simulink model "DiscretizedModel"  (R2023b)
settings: Solver=VariableStepAuto  StartTime=0.0  StopTime=0.5  MaxStep=inverter.param.timeSwitching*0.1  RelTol=1e-3
undefined symbols (not defined in the file or in its folder): contr_D, contr_Q, contr_W, inverter, mot
libraries: eeGeneralControl x1
settings Model: Creator=zambo  LastModifiedBy=zambo

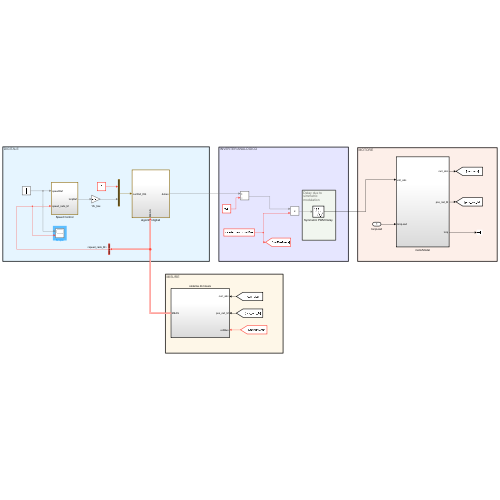
[thumbnail: Simulink's stored preview of the top-level diagram]
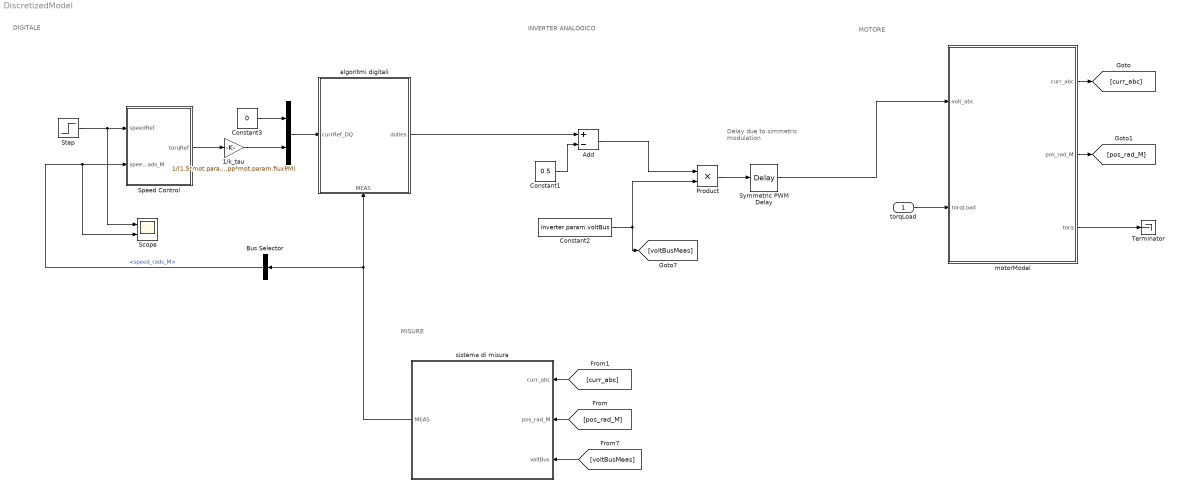
== system DiscretizedModel ==
  note: MISURE
  note: MOTORE
  note: DIGITALE
  note: INVERTER ANALOGICO
  note: Delay due to
      | simmetric
      | modulation
  torqLoad : Inport
  1/k_tau : Gain  Gain=1/(1.5*mot.param.pp*mot.param.fluxPM)
  Add : Sum  Inputs=+-
  Bus Selector : BusSelector  OutputSignals=speed.speed_rads_M
  Constant1 : Constant  Value=0.5  SampleTime=inverter.param.timeSampling
  Constant2 : Constant  Value=inverter.param.voltBus  SampleTime=inverter.param.timeSampling
  Constant3 : Constant  Value=0  SampleTime=inverter.param.timeSampling
  Mux : Mux  Inputs=2
  Product : Product
  Scope : Scope  NumInputPorts=2
  Speed Control : Subsystem
  Step : Step  Time=0.2  After=280  SampleTime=0
  Symmetric PWM Delay : TransportDelay  DelayTime=inverter.param.timeSwitching*0.5
  Terminator : Terminator
  algoritmi digitali : Subsystem
      settings: PortSchema="{\"entries\":[{\"content\":{\"sides\":[{\"content\":{\"connectorIds\":[\"In1\"]},\"type\":\"ConnectorPlacement.EquallySpacedRectSide\",\"uuid\":\"be98b178-87c5-4194-8b79-c3f3cfcc0fc0\"},{\"content\":{\"connectorIds\":[\"Out1\"],\"side\":\"RIGHT\"},\"type\":\"ConnectorPlacement.EquallySpacedRectSide\",\"uuid\":\"8217c3eb-ba2e-412f-a9c4-f2e3b7cd9b00\"},{\"content\":{\"side\":\"TOP\"},\"type\":\"ConnectorPlacement.EquallySpacedRectSide\",\"uuid\":\"9b7fad55-3d61-41f3-9dee-47d3dc8a32f9\"},{\"content\":{\"connectorIds\":[\"In2\"],\"side\":\"BOTTOM\"},\"type\":\"ConnectorPlacement.EquallySpacedRectSide\",\"uuid\":\"8ebbf679-530e-4b8b-8dca-2f31264a1f1b\"}]},\"type\":\"ConnectorPlacement.EquallySpacedConnector\",\"uuid\":\"25d4c349-4b88-4de2-b9c1-687bdffd88d1\"}],\"packageUris\":[\"http://schema.mathworks.com/mf0/Connector/R2020b\"],\"version\":\"1.0\"}"
  motorModel : Subsystem
  sistema di misura : Subsystem
  wires:
  Bus Selector/1 -> Scope/2, Speed Control/2(speed_rads_M)  "<speed_rads_M>"
  Mux/1 -> algoritmi digitali/1(currRef_DQ)
  [pos_rad_M] -> sistema di misura/2(pos_rad_M)
  motorModel/3(torq) -> Terminator/1
  sistema di misura/1(MEAS) -> Bus Selector/1, algoritmi digitali/2(MEAS)
  Step/1 -> Scope/1, Speed Control/1(speedRef)
  [curr_abc] -> sistema di misura/1(curr_abc)
  motorModel/2(pos_rad_M) -> [pos_rad_M]
  Constant1/1 -> Add/2
  Symmetric PWM Delay/1 -> motorModel/1(volt_abc)
  Speed Control/1(torqRef) -> 1/k_tau/1
  Add/1 -> Product/1
  Product/1 -> Symmetric PWM Delay/1
  motorModel/1(curr_abc) -> [curr_abc]
  Constant3/1 -> Mux/1
  algoritmi digitali/1(duties) -> Add/1
  Constant2/1 -> Product/2, [voltBusMeas]
  1/k_tau/1 -> Mux/2
  [voltBusMeas] -> sistema di misura/3(voltBus)
  torqLoad/1 -> motorModel/2(torqLoad)

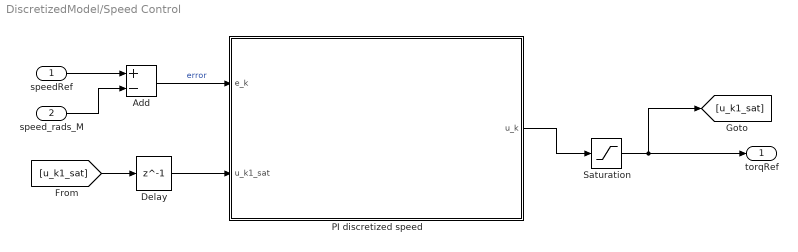
== system DiscretizedModel/Speed Control ==
  speedRef : Inport
  speed_rads_M : Inport  Port=2
  Add : Sum  Inputs=+-
  Delay : Delay  DelayLength=1
  PI discretized speed : MATLAB Function  TreatAsAtomicUnit=on
  Saturation : Saturate  UpperLimit=0.22  LowerLimit=-0.22
  torqRef : Outport
  wires:
  speedRef/1 -> Add/1
  speed_rads_M/1 -> Add/2
  Saturation/1 -> [u_k1_sat], torqRef/1
  Add/1 -> PI discretized speed/1(e_k)  "error"
  PI discretized speed/1(u_k) -> Saturation/1
  [u_k1_sat] -> Delay/1
  Delay/1 -> PI discretized speed/2(u_k1_sat)

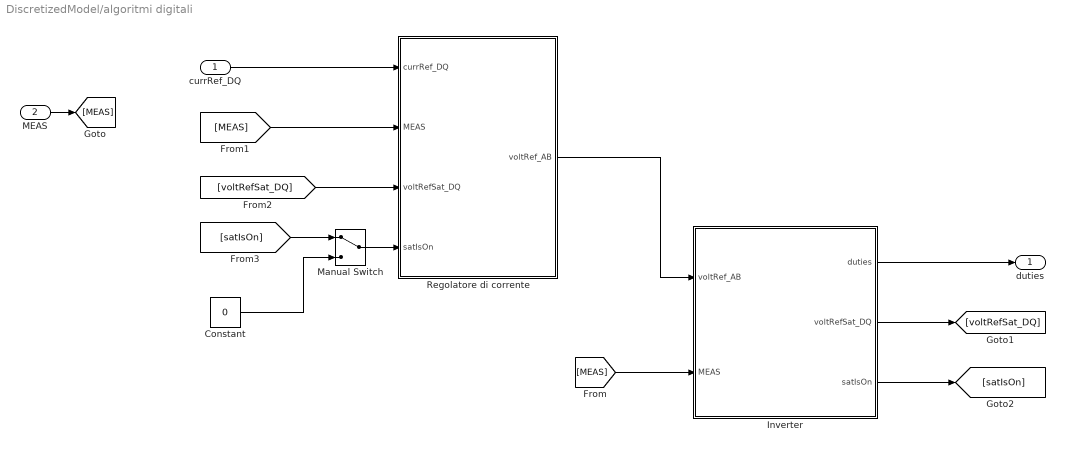
== system DiscretizedModel/algoritmi digitali ==
  currRef_DQ : Inport
  MEAS : Inport  Port=2
  Constant : Constant  Value=0  SampleTime=inverter.param.timeSampling
  Inverter : Subsystem
  Manual Switch : ManualSwitch
  Regolatore di corrente : Subsystem
  duties : Outport
  wires:
  Inverter/1(duties) -> duties/1
  MEAS/1 -> [MEAS]
  [MEAS] -> Inverter/2(MEAS)
  currRef_DQ/1 -> Regolatore di corrente/1(currRef_DQ)
  Regolatore di corrente/1(voltRef_AB) -> Inverter/1(voltRef_AB)
  Inverter/3(satIsOn) -> [satIsOn]
  [MEAS] -> Regolatore di corrente/2(MEAS)
  Inverter/2(voltRefSat_DQ) -> [voltRefSat_DQ]
  [voltRefSat_DQ] -> Regolatore di corrente/3(voltRefSat_DQ)
  Manual Switch/1 -> Regolatore di corrente/4(satIsOn)
  Constant/1 -> Manual Switch/2
  [satIsOn] -> Manual Switch/1

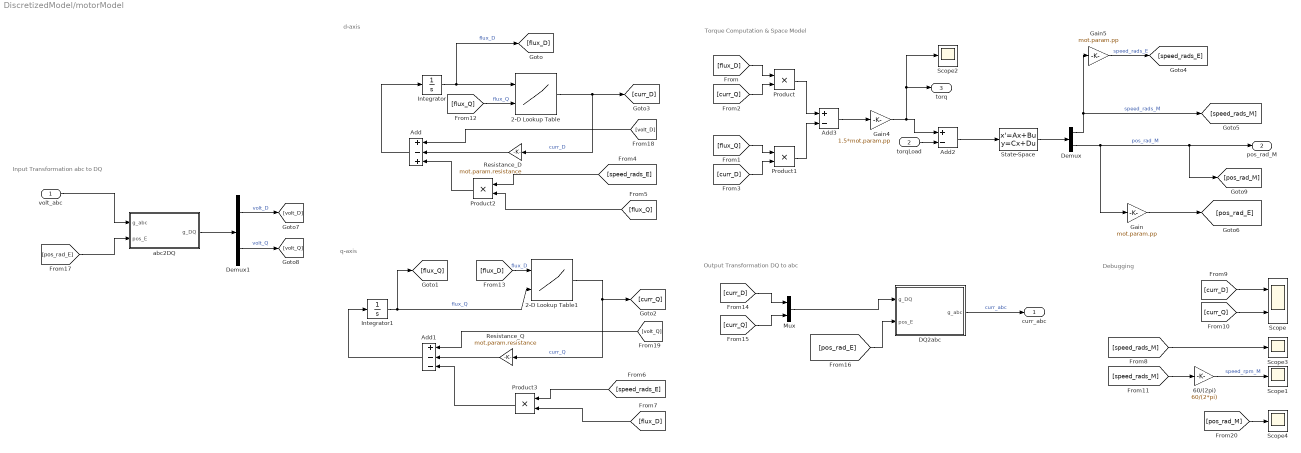
== system DiscretizedModel/motorModel ==
  note: q-axis
  note: d-axis
  note: Debugging
  note: Torque Computation & Space Model
  note: Output Transformation DQ to abc
  note: Input Transformation abc to DQ
  volt_abc : Inport
  torqLoad : Inport  Port=2
  2-D Lookup Table : Lookup_n-D  BreakpointsForDimension1=mot.maps.fluxVec_D  BreakpointsForDimension2=mot.maps.fluxVec_Q  Table=mot.maps.currMap_D'  InternalRulePriority=Speed  RndMeth=Simplest
      settings: InputPortMap=u0,u1
  2-D Lookup Table1 : Lookup_n-D  BreakpointsForDimension1=mot.maps.fluxVec_D  BreakpointsForDimension2=mot.maps.fluxVec_Q  Table=mot.maps.currMap_Q'  InternalRulePriority=Speed  RndMeth=Simplest
      settings: InputPortMap=u0,u1
  60/(2pi) : Gain  Gain=60/(2*pi)
  Add : Sum  Inputs=+-+
  Add1 : Sum  Inputs=+--
  Add2 : Sum  Inputs=+-
  Add3 : Sum  Inputs=+-
  DQ2abc : MATLAB Function  TreatAsAtomicUnit=on
  Demux : Demux  Outputs=2
  Demux1 : Demux  Outputs=2
  Gain : Gain  Gain=mot.param.pp
  Gain4 : Gain  Gain=1.5*mot.param.pp
  Gain5 : Gain  Gain=mot.param.pp
  Integrator : Integrator  InitialCondition=mot.param.fluxPM
  Integrator1 : Integrator
  Mux : Mux  Inputs=2
  Product{,1..3} (4 alike) : Product
  Resistance_D : Gain  Gain=mot.param.resistance
  Resistance_Q : Gain  Gain=mot.param.resistance
  Scope : Scope  NumInputPorts=2
  Scope{1..4} (4 alike) : Scope
  State-Space : StateSpace  A=mot.param.Amech  B=mot.param.Bmech  C=mot.param.Cmech  D=mot.param.Dmech  InitialCondition=[0 0]
  abc2DQ : MATLAB Function  TreatAsAtomicUnit=on
  curr_abc : Outport
  pos_rad_M : Outport  Port=2
  torq : Outport  Port=3
  wires:
  [volt_Q] -> Add1/1
  [flux_Q] -> 2-D Lookup Table/2  "flux_Q"
  [speed_rads_M] -> Scope3/1
  Gain/1 -> [pos_rad_E]
  Integrator/1 -> 2-D Lookup Table/1, [flux_D]  "flux_D"
  [curr_D] -> Mux/1
  Demux1/2 -> [volt_Q]  "volt_Q"
  [pos_rad_E] -> abc2DQ/2(pos_E)
  [curr_Q] -> Product/2
  abc2DQ/1(g_DQ) -> Demux1/1
  Resistance_Q/1 -> Add1/2
  [curr_Q] -> Mux/2
  Product3/1 -> Add1/3
  [pos_rad_E] -> DQ2abc/2(pos_E)
  Demux1/1 -> [volt_D]  "volt_D"
  [flux_D] -> Product3/2
  [speed_rads_E] -> Product2/1
  Demux/2 -> Gain/1, [pos_rad_M], pos_rad_M/1  "pos_rad_M"
  Product2/1 -> Add/3
  [speed_rads_E] -> Product3/1
  Product/1 -> Add3/1
  Add1/1 -> Integrator1/1
  DQ2abc/1(g_abc) -> curr_abc/1  "curr_abc"
  2-D Lookup Table/1 -> Resistance_D/1, [curr_D]  "curr_D"
  Add3/1 -> Gain4/1
  [curr_D] -> Product1/2
  [flux_D] -> Product/1
  Add/1 -> Integrator/1
  Product1/1 -> Add3/2
  volt_abc/1 -> abc2DQ/1(g_abc)
  Integrator1/1 -> 2-D Lookup Table1/2, [flux_Q]  "flux_Q"
  Demux/1 -> [speed_rads_M], Gain5/1  "speed_rads_M"
  [pos_rad_M] -> Scope4/1
  Gain4/1 -> torq/1, Scope2/1, Add2/1
  [speed_rads_M] -> 60/(2pi)/1
  Gain5/1 -> [speed_rads_E]  "speed_rads_E"
  Resistance_D/1 -> Add/2
  2-D Lookup Table1/1 -> Resistance_Q/1, [curr_Q]  "curr_Q"
  60/(2pi)/1 -> Scope1/1  "speed_rpm_M"
  [volt_D] -> Add/1
  [flux_Q] -> Product2/2
  Mux/1 -> DQ2abc/1(g_DQ)
  [curr_D] -> Scope/1
  [flux_Q] -> Product1/1
  State-Space/1 -> Demux/1
  [flux_D] -> 2-D Lookup Table1/1  "flux_D"
  [curr_Q] -> Scope/2
  Add2/1 -> State-Space/1
  torqLoad/1 -> Add2/2

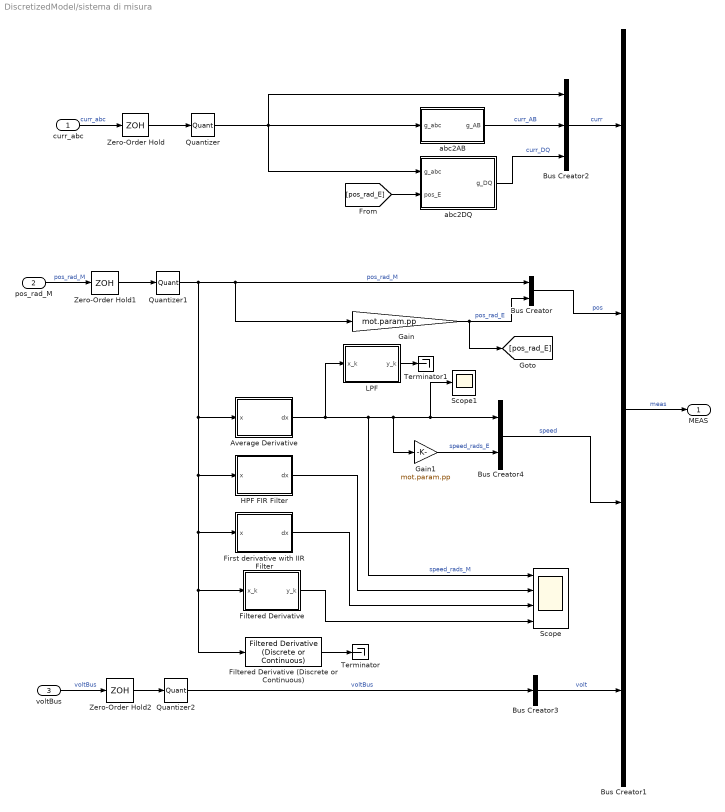
== system DiscretizedModel/sistema di misura ==
  curr_abc : Inport
  pos_rad_M : Inport  Port=2
  voltBus : Inport  Port=3
  Average Derivative : MATLAB Function  TreatAsAtomicUnit=on
  Bus Creator : BusCreator  Inputs=2
  Bus Creator1 : BusCreator  Inputs=4
  Bus Creator2 : BusCreator  Inputs=3
  Bus Creator3 : BusCreator  Inputs=1
  Bus Creator4 : BusCreator  Inputs=2
  Filtered Derivative : MATLAB Function  TreatAsAtomicUnit=on
  Filtered Derivative (Discrete or Continuous) : eeGeneralControl/Filtered Derivative (Discrete or Continuous)  K=1  T=3.9809e-04  B=inf  A=-inf  minRatio=10  init_option=Inherited from block input  x0=0  Ts=inverter.param.timeSampling
      settings: LibrarySourceBlock=|
      | ee_sl_lib/General Control/Filtered Derivative
      | (Discrete or Continuous)
  First derivative with IIR Filter : MATLAB Function  TreatAsAtomicUnit=on
  Gain : Gain  Gain=mot.param.pp
  Gain1 : Gain  Gain=mot.param.pp
  HPF FIR Filter : MATLAB Function  TreatAsAtomicUnit=on
  LPF : MATLAB Function  TreatAsAtomicUnit=on
  Quantizer : Quantizer  QuantizationInterval=meas.quant.currMeas
  Quantizer1 : Quantizer  QuantizationInterval=meas.quant.currMeas
  Quantizer2 : Quantizer  QuantizationInterval=meas.quant.currMeas
  Scope : Scope  NumInputPorts=4
  Scope1 : Scope
  Terminator : Terminator
  Terminator1 : Terminator
  Zero-Order Hold : ZeroOrderHold  SampleTime=inverter.param.timeSampling
  Zero-Order Hold1 : ZeroOrderHold  SampleTime=inverter.param.timeSampling
  Zero-Order Hold2 : ZeroOrderHold  SampleTime=inverter.param.timeSampling
  abc2AB : MATLAB Function  TreatAsAtomicUnit=on
  abc2DQ : MATLAB Function  TreatAsAtomicUnit=on
  MEAS : Outport
  wires:
  Bus Creator2/1 -> Bus Creator1/1  "curr"
  pos_rad_M/1 -> Zero-Order Hold1/1  "pos_rad_M"
  abc2DQ/1(g_DQ) -> Bus Creator2/3  "curr_DQ"
  Gain/1 -> [pos_rad_E], Bus Creator/2  "pos_rad_E"
  Quantizer1/1 -> Filtered Derivative (Discrete or Continuous)/1, Filtered Derivative/1(x_k), First derivative with IIR Filter/1(x), HPF FIR Filter/1(x), Average Derivative/1(x), Gain/1, Bus Creator/1  "pos_rad_M"
  Gain1/1 -> Bus Creator4/2  "speed_rads_E"
  Bus Creator4/1 -> Bus Creator1/3  "speed"
  Zero-Order Hold1/1 -> Quantizer1/1
  curr_abc/1 -> Zero-Order Hold/1  "curr_abc"
  [pos_rad_E] -> abc2DQ/2(pos_E)
  Zero-Order Hold/1 -> Quantizer/1
  Bus Creator1/1 -> MEAS/1  "meas"
  Bus Creator/1 -> Bus Creator1/2  "pos"
  Bus Creator3/1 -> Bus Creator1/4  "volt"
  abc2AB/1(g_AB) -> Bus Creator2/2  "curr_AB"
  Quantizer/1 -> abc2DQ/1(g_abc), Bus Creator2/1, abc2AB/1(g_abc)
  Average Derivative/1(dx) -> LPF/1(x_k), Scope1/1, Bus Creator4/1, Gain1/1, Scope/1  "speed_rads_M"
  Zero-Order Hold2/1 -> Quantizer2/1
  voltBus/1 -> Zero-Order Hold2/1  "voltBus"
  Quantizer2/1 -> Bus Creator3/1  "voltBus"
  First derivative with IIR Filter/1(dx) -> Scope/3
  HPF FIR Filter/1(dx) -> Scope/2
  Filtered Derivative/1(y_k) -> Scope/4
  Filtered Derivative (Discrete or Continuous)/1 -> Terminator/1
  LPF/1(y_k) -> Terminator1/1

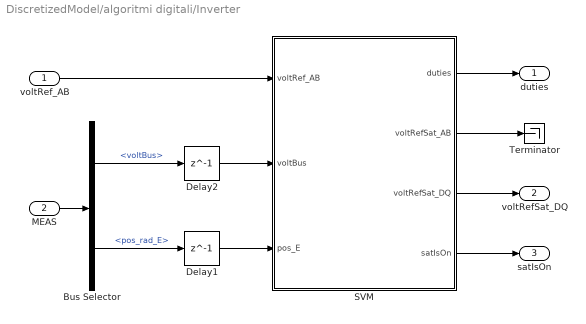
== system DiscretizedModel/algoritmi digitali/Inverter ==
  voltRef_AB : Inport
  MEAS : Inport  Port=2
  Bus Selector : BusSelector  OutputSignals=volt.voltBus,pos.pos_rad_E
  Delay1 : Delay  DelayLength=1
  Delay2 : Delay  DelayLength=1
  SVM : MATLAB Function  TreatAsAtomicUnit=on
  Terminator : Terminator
  duties : Outport
  voltRefSat_DQ : Outport  Port=2
  satIsOn : Outport  Port=3
  wires:
  Bus Selector/2 -> Delay1/1  "<pos_rad_E>"
  Delay1/1 -> SVM/3(pos_E)
  Delay2/1 -> SVM/2(voltBus)
  Bus Selector/1 -> Delay2/1  "<voltBus>"
  MEAS/1 -> Bus Selector/1
  voltRef_AB/1 -> SVM/1(voltRef_AB)
  SVM/1(duties) -> duties/1
  SVM/2(voltRefSat_AB) -> Terminator/1
  SVM/3(voltRefSat_DQ) -> voltRefSat_DQ/1
  SVM/4(satIsOn) -> satIsOn/1

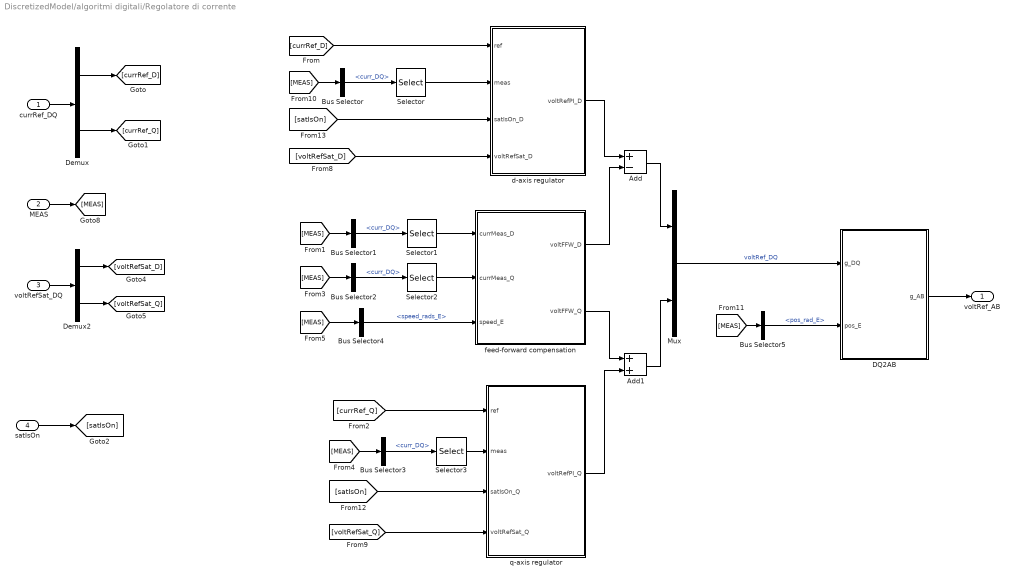
== system DiscretizedModel/algoritmi digitali/Regolatore di corrente ==
  currRef_DQ : Inport
  MEAS : Inport  Port=2
  voltRefSat_DQ : Inport  Port=3
  satIsOn : Inport  Port=4
  Add : Sum  Inputs=+-
  Add1 : Sum
  Bus Selector{,1..3} (4 alike) : BusSelector  OutputSignals=curr.curr_DQ
  Bus Selector4 : BusSelector  OutputSignals=speed.speed_rads_E
  Bus Selector5 : BusSelector  OutputSignals=pos.pos_rad_E
  DQ2AB : MATLAB Function  TreatAsAtomicUnit=on
  Demux : Demux  Outputs=2
  Demux2 : Demux  Outputs=2
  Mux : Mux  Inputs=2
  Selector : Selector  InputPortWidth=2  IndexOptions=Index vector (dialog)  Indices=[1]  OutputSizes=1
  Selector1 : Selector  InputPortWidth=2  IndexOptions=Index vector (dialog)  Indices=[1]  OutputSizes=1
  Selector2 : Selector  InputPortWidth=2  IndexOptions=Index vector (dialog)  Indices=[2]  OutputSizes=1
  Selector3 : Selector  InputPortWidth=2  IndexOptions=Index vector (dialog)  Indices=[2]  OutputSizes=1
  d-axis regulator : Subsystem
  feed-forward compensation : Subsystem
  q-axis regulator : Subsystem
  voltRef_AB : Outport
  wires:
  currRef_DQ/1 -> Demux/1
  voltRefSat_DQ/1 -> Demux2/1
  Demux/1 -> [currRef_D]
  Demux/2 -> [currRef_Q]
  [currRef_D] -> d-axis regulator/1(ref)
  [currRef_Q] -> q-axis regulator/1(ref)
  d-axis regulator/1(voltRefPI_D) -> Add/1
  feed-forward compensation/1(voltFFW_D) -> Add/2
  feed-forward compensation/2(voltFFW_Q) -> Add1/1
  q-axis regulator/1(voltRefPI_Q) -> Add1/2
  Add1/1 -> Mux/2
  Add/1 -> Mux/1
  Demux2/1 -> [voltRefSat_D]
  Demux2/2 -> [voltRefSat_Q]
  [voltRefSat_D] -> d-axis regulator/4(voltRefSat_D)
  [voltRefSat_Q] -> q-axis regulator/4(voltRefSat_Q)
  Mux/1 -> DQ2AB/1(g_DQ)  "voltRef_DQ"
  DQ2AB/1(g_AB) -> voltRef_AB/1
  MEAS/1 -> [MEAS]
  [MEAS] -> Bus Selector/1
  Bus Selector/1 -> Selector/1  "<curr_DQ>"
  Selector/1 -> d-axis regulator/2(meas)
  Bus Selector1/1 -> Selector1/1  "<curr_DQ>"
  [MEAS] -> Bus Selector1/1
  Selector1/1 -> feed-forward compensation/1(currMeas_D)
  [MEAS] -> Bus Selector2/1
  Bus Selector2/1 -> Selector2/1  "<curr_DQ>"
  Selector2/1 -> feed-forward compensation/2(currMeas_Q)
  Bus Selector3/1 -> Selector3/1  "<curr_DQ>"
  [MEAS] -> Bus Selector3/1
  Selector3/1 -> q-axis regulator/2(meas)
  [MEAS] -> Bus Selector4/1
  Bus Selector4/1 -> feed-forward compensation/3(speed_E)  "<speed_rads_E>"
  [MEAS] -> Bus Selector5/1
  Bus Selector5/1 -> DQ2AB/2(pos_E)  "<pos_rad_E>"
  satIsOn/1 -> [satIsOn]
  [satIsOn] -> q-axis regulator/3(satIsOn_Q)
  [satIsOn] -> d-axis regulator/3(satIsOn_D)

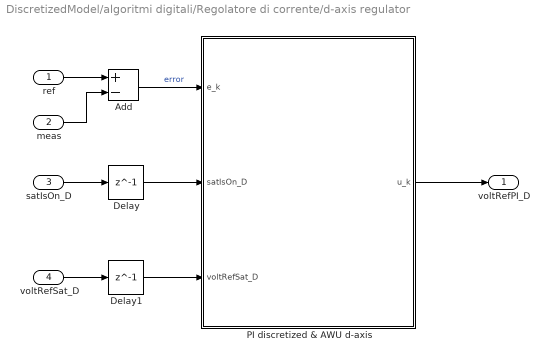
== system DiscretizedModel/algoritmi digitali/Regolatore di corrente/d-axis regulator ==
  ref : Inport
  meas : Inport  Port=2
  satIsOn_D : Inport  Port=3
  voltRefSat_D : Inport  Port=4
  Add : Sum  Inputs=+-
  Delay : Delay  DelayLength=1
  Delay1 : Delay  DelayLength=1
  PI discretized & AWU d-axis : MATLAB Function  TreatAsAtomicUnit=on
  voltRefPI_D : Outport
  wires:
  meas/1 -> Add/2
  ref/1 -> Add/1
  satIsOn_D/1 -> Delay/1
  voltRefSat_D/1 -> Delay1/1
  Add/1 -> PI discretized & AWU d-axis/1(e_k)  "error"
  Delay/1 -> PI discretized & AWU d-axis/2(satIsOn_D)
  Delay1/1 -> PI discretized & AWU d-axis/3(voltRefSat_D)
  PI discretized & AWU d-axis/1(u_k) -> voltRefPI_D/1

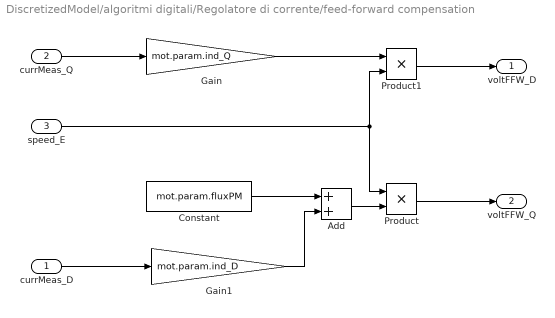
== system DiscretizedModel/algoritmi digitali/Regolatore di corrente/feed-forward compensation ==
  currMeas_D : Inport
  currMeas_Q : Inport  Port=2
  speed_E : Inport  Port=3
  Add : Sum
  Constant : Constant  Value=mot.param.fluxPM
  Gain : Gain  Gain=mot.param.ind_Q
  Gain1 : Gain  Gain=mot.param.ind_D
  Product : Product
  Product1 : Product
  voltFFW_D : Outport
  voltFFW_Q : Outport  Port=2
  wires:
  currMeas_D/1 -> Gain1/1
  currMeas_Q/1 -> Gain/1
  Constant/1 -> Add/1
  Gain1/1 -> Add/2
  Add/1 -> Product/2
  speed_E/1 -> Product/1, Product1/2
  Gain/1 -> Product1/1
  Product1/1 -> voltFFW_D/1
  Product/1 -> voltFFW_Q/1

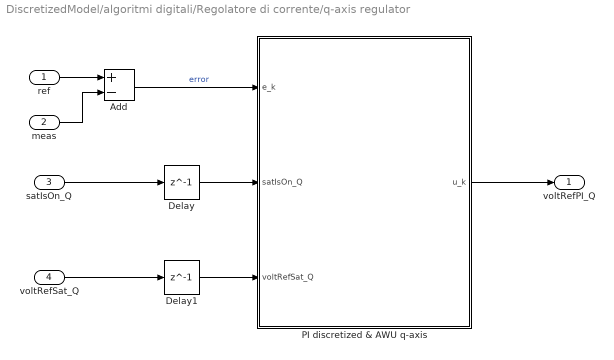
== system DiscretizedModel/algoritmi digitali/Regolatore di corrente/q-axis regulator ==
  ref : Inport
  meas : Inport  Port=2
  satIsOn_Q : Inport  Port=3
  voltRefSat_Q : Inport  Port=4
  Add : Sum  Inputs=+-
  Delay : Delay  DelayLength=1
  Delay1 : Delay  DelayLength=1
  PI discretized & AWU q-axis : MATLAB Function  TreatAsAtomicUnit=on
  voltRefPI_Q : Outport
  wires:
  ref/1 -> Add/1
  meas/1 -> Add/2
  Delay/1 -> PI discretized & AWU q-axis/2(satIsOn_Q)
  Delay1/1 -> PI discretized & AWU q-axis/3(voltRefSat_Q)
  Add/1 -> PI discretized & AWU q-axis/1(e_k)  "error"
  satIsOn_Q/1 -> Delay/1
  voltRefSat_Q/1 -> Delay1/1
  PI discretized & AWU q-axis/1(u_k) -> voltRefPI_Q/1

== matlab function DiscretizedModel/algoritmi digitali/Regolatore di corrente/d-axis regulator/PI discretized & AWU d-axis ==
  data: e_k input; satIsOn_D input; u_k output; voltRefSat_D input; contr_D parameter; inverter parameter
function u_k = fcn(e_k, satIsOn_D, voltRefSat_D, contr_D, inverter)

% Parameters
kp = contr_D.param.propGain;                    % Proportional gain
ki = contr_D.param.intGain;                     % Integral gain
T = inverter.param.timeSampling;                % Sampling period (seconds)

% Initialization
persistent e_k1                                 % Error e(k-1)
persistent yI_k1                                % Integral term yI(k-1)

% Check
if (isempty(e_k1) || isempty (yI_k1))
    e_k1   = 0;
    yI_k1  = 0;
end

% Anti-windup
if ((satIsOn_D == 1) && (((voltRefSat_D < 0) && (e_k > 0)) || ((voltRefSat_D > 0) && (e_k < 0))))
    ki = 0;
end

% Calculate up_k
up_k = kp * e_k;

% Update integral term with anti-windup
yI_k = yI_k1 + ki * e_k1 * T;

% Compute control output
u_k = up_k + yI_k;

% Update persistent variables
yI_k1=yI_k;
e_k1=e_k;


end

== matlab function DiscretizedModel/sistema di misura/HPF FIR Filter ==
  data: x input; dx output; inverter parameter
function dx = fcn(x, inverter)

% Parameters
T       = inverter.param.timeSampling;
n_tabs  = 4;

% Initialize persistent variables
persistent x_k1;      % x(k-1)
persistent x_k2;      % x(k-2)
persistent x_k3;      % x(k-3)
persistent x_k4;      % x(k-4)


% check
if (isempty(x_k1) && isempty(x_k2) && isempty(x_k3))
    x_k1 = 0;
    x_k2 = 0;
    x_k3 = 0;
    x_k4 = 0;
end

% calculate
dx = (x-x_k4)/(n_tabs*T);

% update variables
x_k4 = x_k3;
x_k3 = x_k2;
x_k2 = x_k1;
x_k1 = x;


end

== matlab function DiscretizedModel/sistema di misura/First derivative with IIR Filter ==
  data: x input; dx output; inverter parameter
function dx = fcn(x, inverter)

% Parameters
T       = inverter.param.timeSampling;
fs      = 1/T;
n_tabs  = 4;

tau = 1/(2*pi*fs/n_tabs);
alpha = tau/(tau+T);

% Initialize persistent variables
persistent dx_k1;   % dx(k-1)
persistent x_k1;    % x(k-1)

% check
if (isempty(dx_k1) && isempty(x_k1))
    dx_k1 = 0;
    x_k1 = 0;
end

dx = (1 - alpha) * dx_k1 + alpha / T * (x-x_k1);

% update variables
dx_k1 = dx;
x_k1 = x;

end

== matlab function DiscretizedModel/sistema di misura/LPF ==
  data: x_k input; y_k output
function y_k = fcn(x_k)

b          = 0.9;   % coefficient 
persistent y_k1         % y(k-1)

if isempty(y_k1)
    y_k1=0;
end

% Filtering the input
y_k= b * x_k + (1-b)*y_k1;

% Refresh the variable y(k-1)
y_k1=y_k;

end

== matlab function DiscretizedModel/sistema di misura/Filtered Derivative ==
  data: x_k input; y_k output; inverter parameter
function y_k = fcn(x_k,inverter)

% parameters
Ts  = inverter.param.timeSampling;
ft  = (0.5*inverter.param.freqSwitching)/10;

tau = 1/(2*pi*ft);

alpha = 2/(2 * tau + Ts);
beta  = (Ts - 2 * tau)/(2 * tau + Ts);

% define persistent variables
persistent y_k1;
persistent x_k1;

% check
if isempty(y_k1)
    y_k1 = 0;
end

if isempty(x_k1)
    x_k1 = 0;
end

% algorithm
y_k = alpha * (x_k - x_k1) - beta * y_k1;

% update variables
y_k1 = y_k;
x_k1 = x_k;

end

== matlab function DiscretizedModel/algoritmi digitali/Inverter/SVM ==
  data: voltRef_AB input; voltBus input; pos_E input; duties output; voltRefSat_AB output; voltRefSat_DQ output; satIsOn output; inverter parameter

function [duties, voltRefSat_AB, voltRefSat_DQ, satIsOn] = fcn(voltRef_AB, voltBus,pos_E, inverter)

%% STEP 1
% initialize variables 
duties=ones(3,1)*0.5;
voltRefSat_AB=zeros(2,1);
satIsOn=0;

k=1;    % costante per ridurre Tm e Tm1 nel caso di saturazione circolare
k1=1;   % costante per ridurre Tm e Tm1 nel caso di saturazione esagonale
m=0;
Tm=0;
Tm1=0;
T0=0;

% define constant
c=1/sqrt(3);


% if cascade to find m
if voltRef_AB(2,1)>0.0
    if abs(voltRef_AB(1,1))>abs(voltRef_AB(2,1)*c)
        if voltRef_AB(1,1)>0.0
            m=1;
        else
            m=3;
        end
    else
        m=2;
    end
else
    if abs(voltRef_AB(1,1))>abs(voltRef_AB(2,1)*c)
        if voltRef_AB(1,1)>0.0
            m=6;
        else
            m=4;
        end
    else
        m=5;
    end
end

%% STEP 2
% Define another constant
c1=sqrt(3)*inverter.param.timeSwitching;

% circle saturation
if (inverter.param.satCircleOn==1)
    if (voltRef_AB(1,1)^2+voltRef_AB(2,1)^2)>((voltBus*c)^2)
        satIsOn=1;
        k=(voltBus*c)/(sqrt(voltRef_AB(1,1)^2+voltRef_AB(2,1)^2));
        voltRefSat_AB=k*voltRef_AB;
    end
end

if (voltBus > 0.2)
    if (satIsOn==1)
        Tm=(c1/voltBus)*(voltRefSat_AB(1,1)*sin(m*(pi/3))-voltRefSat_AB(2,1)*cos(m*(pi/3)));
        Tm1=(c1/voltBus)*(-voltRefSat_AB(1,1)*sin((m-1)*(pi/3))+voltRefSat_AB(2,1)*cos((m-1)*(pi/3)));
        T0=inverter.param.timeSwitching-Tm-Tm1;
    else
        Tm=(c1/voltBus)*(voltRef_AB(1,1)*sin(m*(pi/3))-voltRef_AB(2,1)*cos(m*(pi/3)));
        Tm1=(c1/voltBus)*(-voltRef_AB(1,1)*sin((m-1)*(pi/3))+voltRef_AB(2,1)*cos((m-1)*(pi/3)));
        T0=inverter.param.timeSwitching-Tm-Tm1;
    end
end

%% STEP 3
if (Tm+Tm1 > inverter.param.timeSwitching)
    satIsOn=1;
    k1=inverter.param.timeSwitching/(Tm+Tm1);
    Tm=k1*Tm;
    Tm1=k1*Tm1;
    T0=0;
    voltRefSat_AB=k1*voltRef_AB;
end

%% STEP 4

switch m
    case 1
        duties(1,1)=(Tm+Tm1+T0/2)*inverter.param.freqSwitching;
        duties(2,1)=(Tm1+T0/2)*inverter.param.freqSwitching;
        duties(3,1)=(T0/2)*inverter.param.freqSwitching;
    case 2
        duties(1,1)=(Tm+T0/2)*inverter.param.freqSwitching;
        duties(2,1)=(Tm+Tm1+T0/2)*inverter.param.freqSwitching;
        duties(3,1)=(T0/2)*inverter.param.freqSwitching;
    case 3
        duties(1,1)=(T0/2)*inverter.param.freqSwitching;
        duties(2,1)=(Tm+Tm1+T0/2)*inverter.param.freqSwitching;
        duties(3,1)=(Tm1+T0/2)*inverter.param.freqSwitching;
    case 4
        duties(1,1)=(T0/2)*inverter.param.freqSwitching;
        duties(2,1)=(Tm+T0/2)*inverter.param.freqSwitching;
        duties(3,1)=(Tm+Tm1+T0/2)*inverter.param.freqSwitching;
    case 5
        duties(1,1)=(Tm1+T0/2)*inverter.param.freqSwitching;
        duties(2,1)=(T0/2)*inverter.param.freqSwitching;
        duties(3,1)=(Tm+Tm1+T0/2)*inverter.param.freqSwitching;
    case 6
        duties(1,1)=(Tm+Tm1+T0/2)*inverter.param.freqSwitching;
        duties(2,1)=(T0/2)*inverter.param.freqSwitching;
        duties(3,1)=(Tm+T0/2)*inverter.param.freqSwitching;
    otherwise
        duties(1,1)=0.5;
        duties(2,1)=0.5;
        duties(3,1)=0.5;
end

voltRefSat_DQ = AB2DQ(voltRefSat_AB, pos_E);

end

== matlab function DiscretizedModel/motorModel/DQ2abc ==
  data: g_DQ input; g_abc output; pos_E input
function g_abc = fcn(g_DQ,pos_E)

g_abc   = DQ2abc(g_DQ,pos_E);

end

== matlab function DiscretizedModel/motorModel/abc2DQ ==
  data: g_abc input; g_DQ output; pos_E input
function g_DQ = fcn(g_abc, pos_E)

g_DQ    = abc2DQ(g_abc, pos_E);

end

== matlab function DiscretizedModel/algoritmi digitali/Regolatore di corrente/q-axis regulator/PI discretized & AWU q-axis ==
  data: e_k input; satIsOn_Q input; u_k output; voltRefSat_Q input; contr_Q parameter; inverter parameter
function u_k = fcn(e_k, satIsOn_Q, voltRefSat_Q, contr_Q, inverter)

% Parameters
kp = contr_Q.param.propGain;                    % Proportional gain
ki = contr_Q.param.intGain;                     % Integral gain
T = inverter.param.timeSampling;                % Sampling period (seconds)

% Initialization
persistent e_k1                                 % Error e(k-1)
persistent yI_k1                                % Integral term yI(k-1)

% Check
if (isempty(e_k1) || isempty (yI_k1))
    e_k1   = 0;
    yI_k1  = 0;
end

% Anti-windup
if ((satIsOn_Q == 1) && (((voltRefSat_Q < 0) && (e_k > 0)) || ((voltRefSat_Q > 0) && (e_k < 0))))
    ki = 0;
end

% Calculate up_k
up_k = kp * e_k;

% Update integral term with anti-windup
yI_k = yI_k1 + ki * e_k1 * T;

% Compute control output
u_k = up_k + yI_k;

% Update persistent variables
yI_k1=yI_k;
e_k1=e_k;


end

== matlab function DiscretizedModel/sistema di misura/abc2AB ==
  data: g_abc input; g_AB output
function g_AB = fcn(g_abc)

g_AB    = abc2AB(g_abc);

end

== matlab function DiscretizedModel/sistema di misura/abc2DQ ==
  data: g_abc input; g_DQ output; pos_E input
function g_DQ = fcn(g_abc, pos_E)

g_DQ    = abc2DQ(g_abc, pos_E);

end

== matlab function DiscretizedModel/Speed Control/PI discretized speed ==
  data: e_k input; u_k output; u_k1_sat input; contr_W parameter; inverter parameter
function u_k = fcn(e_k, u_k1_sat, contr_W, inverter)

% Parameters
kp = contr_W.param.propGain;                    % Proportional gain
ki = contr_W.param.intGain;                     % Integral gain
T = inverter.param.timeSampling;                % Sampling period (seconds)

% Initialization
persistent e_k1                                 % Error e(k-1)
persistent yI_k1                                % Integral term yI(k-1)
persistent u_k1                                 % Output u(k-1)

% Check
if (isempty(e_k1))
    e_k1 = 0;
    yI_k1 = 0;
    u_k1 = 0;
end

% Calculate up_k
up_k = kp * e_k;

% Update integral term 
yI_k = ki * T * e_k1 + yI_k1 + T*contr_W.speedContr_kt*(u_k1 - u_k1_sat);

% Compute control output
u_k = up_k + yI_k;

% Update persistent variables
yI_k1 = yI_k;
u_k1  = u_k;
e_k1  = e_k;

end

== matlab function DiscretizedModel/sistema di misura/Average Derivative ==
  data: x input; dx output; inverter parameter
function dx = fcn(x, inverter)

% Parameters
T = inverter.param.timeSampling;

% Initialize persistent variables
persistent x_k1;      % x(k-1)
persistent x_k2;      % x(k-2)
persistent x_k3;      % x(k-3)

% check
if (isempty(x_k1) && isempty(x_k2) && isempty(x_k3))
    x_k1 = 0;
    x_k2 = 0;
    x_k3 = 0;
end

% calculate
dx = (x + 3*x_k1 - 3*x_k2 - x_k3)/(6*T);

% update variables
x_k3 = x_k2;
x_k2 = x_k1;
x_k1 = x;


end

== matlab function DiscretizedModel/algoritmi digitali/Regolatore di corrente/DQ2AB ==
  data: g_DQ input; g_AB output; pos_E input
function g_AB = fcn(g_DQ,pos_E)

g_AB   = DQ2AB(g_DQ,pos_E);

end
